simulink model "ballandbeam"  (R2012b)
settings: Solver=ode45  StartTime=0.0  StopTime=10.0  RelTol=1e-3
values from neighbouring files (symbols this model uses):
  a = theta(i)    [animation.m]    (also in constants.m = 0.7143; overlap.m = b*(ycross-h)/ycross)
  b = 0    [calculateBelonging.m]    (also in constants.m = 9.81; overlap.m = L(3)-R(1))
settings Model: Creator=vsnikkil  LastModifiedBy=vesa

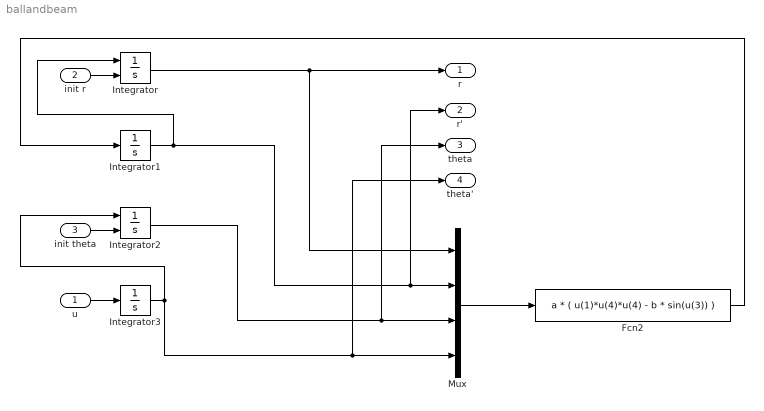
== system ballandbeam ==
  u : Inport
  init r : Inport  Port=2
  init theta : Inport  Port=3
  Fcn2 : Fcn  Expr=a * ( u(1)*u(4)*u(4) - b * sin(u(3)) )
  Integrator : Integrator  InitialConditionSource=external
  Integrator1 : Integrator
  Integrator2 : Integrator  InitialConditionSource=external
  Integrator3 : Integrator
  Mux : Mux
  r : Outport
  r' : Outport  Port=2
  theta : Outport  Port=3
  theta' : Outport  Port=4
  wires:
  Integrator1/1 -> Integrator/1, r'/1, Mux/2
  Integrator3/1 -> theta'/1, Mux/4, Integrator2/1
  Mux/1 -> Fcn2/1
  Integrator/1 -> r/1, Mux/1
  Integrator2/1 -> theta/1, Mux/3
  Fcn2/1 -> Integrator1/1
  init r/1 -> Integrator/2
  init theta/1 -> Integrator2/2
  u/1 -> Integrator3/1
